simulink model "linearLong"  (R2021b)
settings: Solver=VariableStepAuto  StartTime=0.0  StopTime=30  RelTol=1e-3
libraries: slpidlib x2
settings Model: Creator=pablo  LastModifiedBy=jakub
settings SolverCC: AlgebraicLoopSolver=TrustRegion
settings DebuggingCC: SFMachineParentedDataDiag=warning

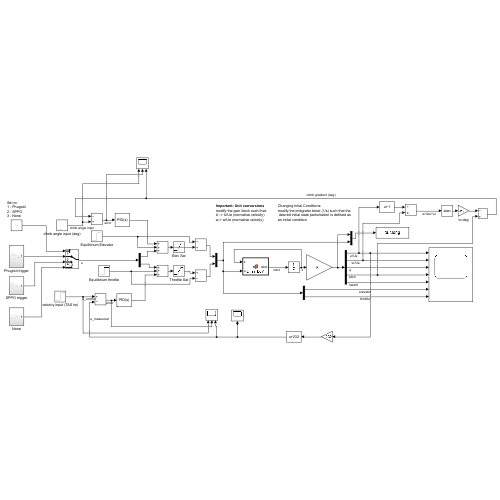
[thumbnail: Simulink's stored preview of the top-level diagram]
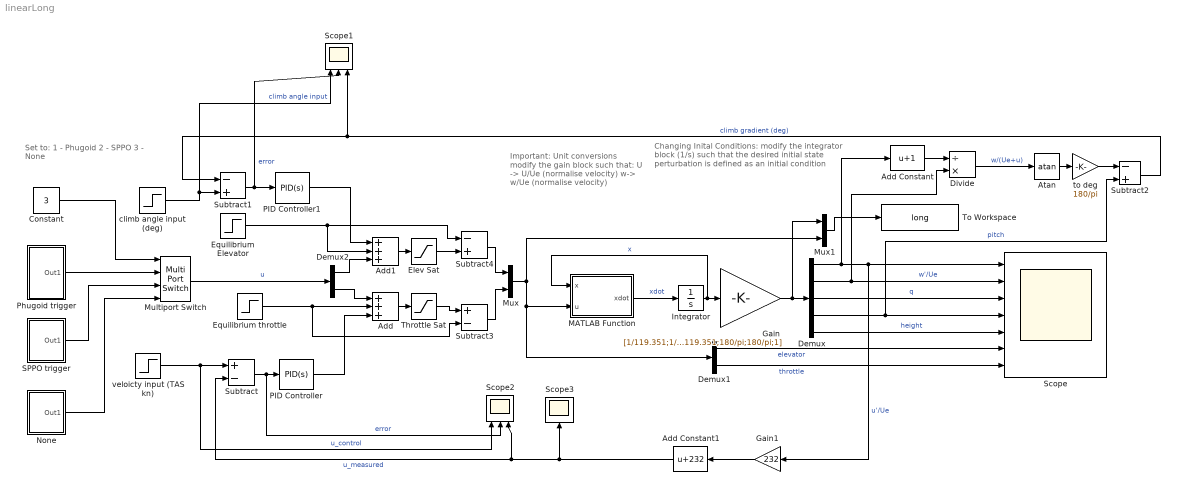
== system linearLong ==
  note: Important: Unit conversions
      | modify the gain block such that:
      | U -> U/Ue (normalise velocity)
      | w-> w/Ue (normalise velocity)
  note: Set to:
      | 1 - Phugoid
      | 2 - SPPO
      | 3 - None
  note: Changing Inital Conditions:
      | modify the integrator block (1/s) such that the
      | desired initial state perturbation is defined as
      | an initial condition
  Add : Sum  Inputs=+++
  Add Constant : Bias  Bias=1
  Add Constant1 : Bias  Bias=232
  Add1 : Sum  Inputs=+++
  Atan : Trigonometry  Operator=atan
  Constant : Constant  Value=3
  Demux : Demux  Outputs=5
  Demux1 : Demux  Outputs=2
  Demux2 : Demux  Outputs=2
  Divide : Product  Inputs=/*
  Elev Sat : Saturate  UpperLimit=1  LowerLimit=-2
  Equilibrium Elevator : Step  SampleTime=0
  Equilibrium throttle : Step  Time=0  After=0.1790  SampleTime=0
  Gain : Gain  Gain=[1/119.351;1/119.351;180/pi;180/pi;1]
  Gain1 : Gain  Gain=232
  Integrator : Integrator  InitialCondition=[0;0;0;0;0]
  MATLAB Function : MATLAB Function  TreatAsAtomicUnit=on
  Multiport Switch : MultiPortSwitch
  Mux : Mux  Inputs=2
  Mux1 : Mux  Inputs=2
  None : Subsystem
  PID Controller : slpidlib/PID Controller  Controller=PID  Form=Parallel  TimeDomain=Continuous-time  UseExternalTs=off  SampleTime=-1  IntegratorMethod=Forward Euler  FilterMethod=Forward Euler  ControllerParametersSource=internal  P=0  I=0  D=0  UseFilter=on  N=100  TunerSelectOption=Transfer Function Based (PID Tuner App)  InitialConditionSource=internal  InitialConditionForIntegrator=0  InitialConditionForFilter=0  DifferentiatorICPrevScaledInput=0  ExternalReset=none  TrackingMode=off  Kt=1  LimitOutput=off  SatLimitsSource=internal  UpperSaturationLimit=inf  LowerSaturationLimit=-inf  LinearizeAsGain=on  AntiWindupMode=none  Kb=1  POutMin=[]  POutMax=[]  IOutMin=[]  IOutMax=[]  DOutMin=[]  DOutMax=[]  NOutMin=[]  NOutMax=[]  SumOutMin=[]  SumOutMax=[]  SaturationOutMin=[]  SaturationOutMax=[]  PParamMin=[]  PParamMax=[]  IParamMin=[]  IParamMax=[]  DParamMin=[]  DParamMax=[]  NParamMin=[]  NParamMax=[]  KbParamMin=[]  KbParamMax=[]  KtParamMin=[]  KtParamMax=[]  KbOutMin=[]  KbOutMax=[]  KtOutMin=[]  KtOutMax=[]  IntegratorOutMin=[]  IntegratorOutMax=[]  FilterOutMin=[]  FilterOutMax=[]  SumI1OutMin=[]  SumI1OutMax=[]  SumI2OutMin=[]  SumI2OutMax=[]  SumI3OutMin=[]  SumI3OutMax=[]  SumI4OutMin=[]  SumI4OutMax=[]  SumDOutMin=[]  SumDOutMax=[]  DifferentiatorOutMin=[]  DifferentiatorOutMax=[]  FilterDiffOutCoefMin=[]  FilterDiffOutCoefMax=[]  ReciprocalOutMin=[]  ReciprocalOutMax=[]  SumDenOutMin=[]  SumDenOutMax=[]  SumNumOutMin=[]  SumNumOutMax=[]  DivideOutMin=[]  DivideOutMax=[]  UdiffTsProdOutMin=[]  UdiffTsProdOutMax=[]  NTsProdOutMin=[]  NTsProdOutMax=[]  UintegralTsProdOutMin=[]  UintegralTsProdOutMax=[]  UngainTsProdOutMin=[]  UngainTsProdOutMax=[]  IntegratorContinuousStateAttributes=''  IntegratorStateMustResolveToSignalObject=off  IntegratorRTWStateStorageClass=Auto  FilterContinuousStateAttributes=''  FilterStateMustResolveToSignalObject=off  FilterRTWStateStorageClass=Auto  ParallelPVariant=InternalParameters  IdealPVariant=Disabled  IVariant=InternalParameters  DVariant=InternalParameters  IntegratorVariant=Continuous  SatVariant=Disabled  AWVariant=Passthrough  PCopyVariant=Disabled  TRVariant=Disabled  FdbkBlocksVariant=Forward  IdealPFdbkVariant=Disabled  SatFdbkVariant=Disabled  DerivativeFilterVariant=ContFilter  NVariant=InternalParameters  NCopyVariant=Disabled  FilterICVariant=InternalICsFilter  IntegratorICVariant=InternalICs  ExternalResetVariant=Disabled  TRSumVariant=Passthrough  SumFdbkVariant=Disabled  SumVariant=Sum_PID  TsampFilterVariant=InternalTs  TsampNgainVariant=Passthrough  TsampIntegralVariant=Passthrough  ExternalSaturationOutDataTypeStr=Inherit: Same as second input
  PID Controller1 : slpidlib/PID Controller  Controller=PID  Form=Parallel  TimeDomain=Continuous-time  UseExternalTs=off  SampleTime=-1  IntegratorMethod=Forward Euler  FilterMethod=Forward Euler  ControllerParametersSource=internal  P=-0.1  I=-0.03  D=0  UseFilter=on  N=100  TunerSelectOption=Transfer Function Based (PID Tuner App)  InitialConditionSource=internal  InitialConditionForIntegrator=0  InitialConditionForFilter=0  DifferentiatorICPrevScaledInput=0  ExternalReset=none  TrackingMode=off  Kt=1  LimitOutput=off  SatLimitsSource=internal  UpperSaturationLimit=inf  LowerSaturationLimit=-inf  LinearizeAsGain=on  AntiWindupMode=none  Kb=1  POutMin=[]  POutMax=[]  IOutMin=[]  IOutMax=[]  DOutMin=[]  DOutMax=[]  NOutMin=[]  NOutMax=[]  SumOutMin=[]  SumOutMax=[]  SaturationOutMin=[]  SaturationOutMax=[]  PParamMin=[]  PParamMax=[]  IParamMin=[]  IParamMax=[]  DParamMin=[]  DParamMax=[]  NParamMin=[]  NParamMax=[]  KbParamMin=[]  KbParamMax=[]  KtParamMin=[]  KtParamMax=[]  KbOutMin=[]  KbOutMax=[]  KtOutMin=[]  KtOutMax=[]  IntegratorOutMin=[]  IntegratorOutMax=[]  FilterOutMin=[]  FilterOutMax=[]  SumI1OutMin=[]  SumI1OutMax=[]  SumI2OutMin=[]  SumI2OutMax=[]  SumI3OutMin=[]  SumI3OutMax=[]  SumI4OutMin=[]  SumI4OutMax=[]  SumDOutMin=[]  SumDOutMax=[]  DifferentiatorOutMin=[]  DifferentiatorOutMax=[]  FilterDiffOutCoefMin=[]  FilterDiffOutCoefMax=[]  ReciprocalOutMin=[]  ReciprocalOutMax=[]  SumDenOutMin=[]  SumDenOutMax=[]  SumNumOutMin=[]  SumNumOutMax=[]  DivideOutMin=[]  DivideOutMax=[]  UdiffTsProdOutMin=[]  UdiffTsProdOutMax=[]  NTsProdOutMin=[]  NTsProdOutMax=[]  UintegralTsProdOutMin=[]  UintegralTsProdOutMax=[]  UngainTsProdOutMin=[]  UngainTsProdOutMax=[]  IntegratorContinuousStateAttributes=''  IntegratorStateMustResolveToSignalObject=off  IntegratorRTWStateStorageClass=Auto  FilterContinuousStateAttributes=''  FilterStateMustResolveToSignalObject=off  FilterRTWStateStorageClass=Auto  ParallelPVariant=InternalParameters  IdealPVariant=Disabled  IVariant=InternalParameters  DVariant=InternalParameters  IntegratorVariant=Continuous  SatVariant=Disabled  AWVariant=Passthrough  PCopyVariant=Disabled  TRVariant=Disabled  FdbkBlocksVariant=Forward  IdealPFdbkVariant=Disabled  SatFdbkVariant=Disabled  DerivativeFilterVariant=ContFilter  NVariant=InternalParameters  NCopyVariant=Disabled  FilterICVariant=InternalICsFilter  IntegratorICVariant=InternalICs  ExternalResetVariant=Disabled  TRSumVariant=Passthrough  SumFdbkVariant=Disabled  SumVariant=Sum_PID  TsampFilterVariant=InternalTs  TsampNgainVariant=Passthrough  TsampIntegralVariant=Passthrough  ExternalSaturationOutDataTypeStr=Inherit: Same as second input
  Phugoid trigger : Subsystem
  SPPO trigger : Subsystem
  Scope : Scope  NumInputPorts=7
  Scope1 : Scope  NumInputPorts=3
  Scope2 : Scope  NumInputPorts=3
  Scope3 : Scope
  Subtract : Sum  Inputs=+-
  Subtract1 : Sum  Inputs=-+
  Subtract2 : Sum  Inputs=-+
  Subtract3 : Sum  Inputs=+-
  Subtract4 : Sum  Inputs=-+
  Throttle Sat : Saturate  UpperLimit=1  LowerLimit=0
  To Workspace : ToWorkspace  VariableName=long  SaveFormat=Timeseries  SampleTime=0.01
  climb angle input (deg) : Step  Time=0  After=5  SampleTime=0
  to deg : Gain  Gain=180/pi
  veloicty input (TAS kn) : Step  Time=0  After=240  SampleTime=0
  wires:
  MATLAB Function/1(xdot) -> Integrator/1  "xdot"
  Integrator/1 -> MATLAB Function/1(x), Gain/1  "x"
  Gain/1 -> Mux1/1, Demux/1
  Demux/1 -> Add Constant/1, Gain1/1, Scope/1  "u'/Ue"
  Demux/2 -> Divide/2, Scope/2  "w'/Ue"
  Demux/3 -> Scope/3  "q"
  Demux/4 -> Subtract2/2, Scope/4  "pitch"
  Phugoid trigger/1(Out1) -> Multiport Switch/2
  SPPO trigger/1(Out1) -> Multiport Switch/3
  Demux1/1 -> Scope/6  "elevator"
  Demux1/2 -> Scope/7  "throttle"
  Mux1/1 -> To Workspace/1
  Demux/5 -> Scope/5  "height"
  Constant/1 -> Multiport Switch/1
  None/1(Out1) -> Multiport Switch/4
  Demux2/1 -> Add1/3
  Multiport Switch/1 -> Demux2/1  "u"
  Mux/1 -> Mux1/2, Demux1/1, MATLAB Function/2(u)
  Subtract3/1 -> Mux/2
  Demux2/2 -> Add/1
  Add/1 -> Throttle Sat/1
  Add1/1 -> Elev Sat/1
  PID Controller/1 -> Add/3
  Subtract/1 -> Scope2/2, PID Controller/1  "error"
  veloicty input (TAS kn)/1 -> Subtract/1, Scope2/1  "u_control"
  Gain1/1 -> Add Constant1/1
  PID Controller1/1 -> Add1/1
  Subtract1/1 -> PID Controller1/1, Scope1/2  "error"
  climb angle input (deg)/1 -> Subtract1/2, Scope1/1  "climb angle input"
  Add Constant/1 -> Divide/1
  Divide/1 -> Atan/1  "w/(Ue+u)"
  Atan/1 -> to deg/1
  to deg/1 -> Subtract2/1
  Subtract2/1 -> Scope1/3, Subtract1/1  "climb gradient (deg)"
  Add Constant1/1 -> Scope3/1, Scope2/3, Subtract/2  "u_measured"
  Equilibrium throttle/1 -> Add/2, Subtract3/2
  Throttle Sat/1 -> Subtract3/1
  Equilibrium Elevator/1 -> Subtract4/1, Add1/2
  Elev Sat/1 -> Subtract4/2
  Subtract4/1 -> Mux/1

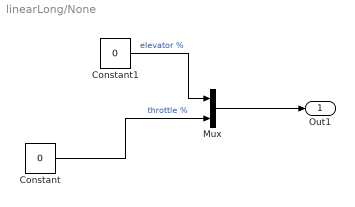
== system linearLong/None ==
  Constant : Constant  Value=0
  Constant1 : Constant  Value=0
  Mux : Mux  Inputs=2
  Out1 : Outport
  wires:
  Constant1/1 -> Mux/1  "elevator %"
  Constant/1 -> Mux/2  "throttle %"
  Mux/1 -> Out1/1

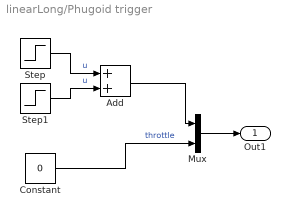
== system linearLong/Phugoid trigger ==
  Add : Sum
  Constant : Constant  Value=0
  Mux : Mux  Inputs=2
  Step : Step  Time=0  After=0.7639  SampleTime=0
  Step1 : Step  Time=0.1  After=-0.7639  SampleTime=0
  Out1 : Outport
  wires:
  Add/1 -> Mux/1
  Step1/1 -> Add/2  "u"
  Step/1 -> Add/1  "u"
  Constant/1 -> Mux/2  "throttle"
  Mux/1 -> Out1/1

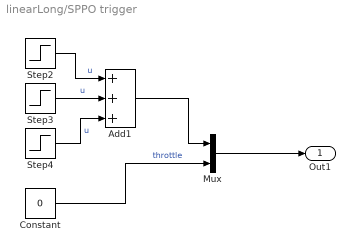
== system linearLong/SPPO trigger ==
  Add1 : Sum  Inputs=+++
  Constant : Constant  Value=0
  Mux : Mux  Inputs=2
  Step2 : Step  Time=0  SampleTime=0
  Step3 : Step  Time=0.1  After=-2  SampleTime=0
  Step4 : Step  Time=0.2  SampleTime=0
  Out1 : Outport
  wires:
  Step4/1 -> Add1/3  "u"
  Step3/1 -> Add1/2  "u"
  Step2/1 -> Add1/1  "u"
  Add1/1 -> Mux/1
  Constant/1 -> Mux/2  "throttle"
  Mux/1 -> Out1/1

== matlab function linearLong/MATLAB Function ==
  data: x input; u input; xdot output
function xdot = LinearEoM(x,u)
%Input: - x:Longitudinal state vactor (5x1 vector)
%         x(1)- u      m/s
%         x(2)- w      m/s
%         x(3)- q      rad/s
%         x(4)- theta  deg
%         x(5)- height m
%       - u: longitudinal control vector (2x1 vector)
%         u(1)- elevator deflection as percentage of max +ve defrlaction
%               -2<u(1)<1     
%         u(2)- Thrust as % of max thrust
%Output: - xdot: (5x1 vector)

%General aircraft parameters
m       =9.2700e+03;      %Mass of aircraft in Kg
Iyy     = 1.1726e+05;      %Kg m^2
g=9.81; %m/s^2
Ue = 114.7211; %m/s

%stability derivatives
%U derivatives
Xu = -115.1871; %Ns/m 
Zu = -1.5854e+03; %Ns/m 
Mu = 0; %Ns 
Xw = 462.5567;  %Ns/m 
Zw = -1.4377e+04;   %Ns/m 
Mw = -9.0429e+03;   %Ns 
Xq = 805.3536;  %Ns 
Zq = -3.3544e+04;   %Ns 
Mq = -2.7467e+05;   %Nms 
Xwdot = 0;  %Ns^2/m - assume effect minimal
Zwdot = -183.8563;  %Ns^2/m 
Mwdot = -1.5055e+03;    %Ns^2 

%Control derivatives 
XiH = -1.5560e+04;  %N/rad
ZiH = -4.7379e+05;  %N/rad
MiH = -3.7853e+06;  %N/rad
%Control derivatives for the throttle
Xt  = 1; %N 
Zt  = 0; %N
Mt  = -0.2800; %Nm

% HELLO
theta_e = 0;
% BYE

A = [Xu/m,Xw/m,0,-g*cos(theta_e),0;
    Zu/(m-Zwdot),Zw/(m-Zwdot),(Zq+m*Ue)/(m-Zwdot),-m*g*sin(theta_e)/(m-Zwdot),0;
    (Mu + Mwdot*Zu/(m-Zwdot))/Iyy,(Mw + Mwdot*Zw/(m-Zwdot))/Iyy,...
    (Mq + Mwdot*(Zq+m*Ue)/(m-Zwdot))/Iyy,-Mwdot*m*g*sin(theta_e)/(Iyy*(m-Zwdot)),0;
    0,0,1,0,0;...
    0,-1,0,Ue,0];
B = [XiH/m,Xt/m;
    ZiH/(m-Zwdot),Zt/(m-Zwdot);
    MiH/Iyy+Mwdot*ZiH/(Iyy*(m-Zwdot)),Mt/Iyy+Mwdot*Zt/(Iyy*(m-Zwdot));
    0,0;
    0,0];

% M = [   m,      -Xwdot,   0,      0,    0;
%         0,      m-Zwdot,  0,      0,    0;
%         0,      -Mwdot,   Iyy,    0,    0;
%         0       0,          0,      1,  0;
%         0,      0,          0,      0,  1];
% 
% A = [  Xu,    Xw,    Xq,    -m*g,   0;
%         Zu,    Zw,    Zq+m*Ue,0,    0;
%         Mu,    Mw,    Mq,    0,     0;
%         0,      0,      1,      0,  0;
%         0,      -1,     0,      Ue, 0];

% B = [   XiH,    Xt;
%         ZiH,    Zt;
%         MiH,    Mt;
%         0,      0;
%         0,      0];

u(1)=u(1)*5*pi/180;
u(2)=u(2)*2*18454;
xdot = A*x + B*u;
% xdot = M\(A*x + B*u);
